simulink model "RGB2YCbCr"  (R2018a)
settings: Solver=VariableStepAuto  StartTime=0.0  StopTime=inf  RelTol=1e-3
InitFcn:
  | height = str2num(get_param([bdroot, '/Image Properties'], 'height'));
  | width = str2num(get_param([bdroot, '/Image Properties'], 'width'));
  | I = imresize(eval(get_param([bdroot, '/Image Properties'], 'image')), [(height) (width)]);
  | I = padarray(I, [1 1], 'replicate');
  | % Change input array to RBG
  | inarray = uint32(double(I(:,:,1))*2^16 + double(I(:,:,3))*2^8 + double(I(:,:,2)));
StopFcn:
  | Out = permute(reshape(simout, [3 width height]), [3 2 1]);
  | imtool(Out);
libraries: xbsIndex_r4 x82, hdlsllib x8, simulink x5, dspsrcs4 x1
settings Model: Creator=rgb11127  LastModifiedBy=Adrian

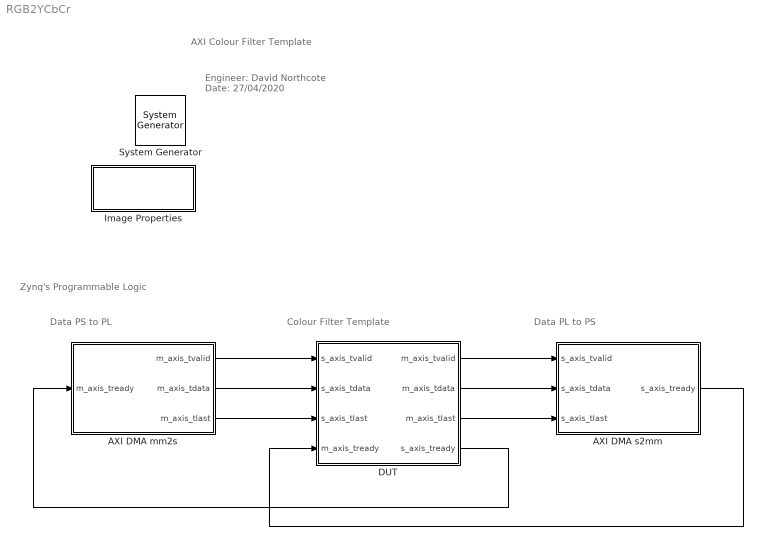
== system RGB2YCbCr ==
  note: Engineer:	David Northcote
      | Date:		27/04/2020
  note: AXI Colour Filter Template
  note: Zynq's Programmable Logic
  note: Data PS to PL
  note: Colour Filter Template
  note: Data PL to PS
  " System Generator" : xbsIndex_r4/ System Generator  Tag=genX  xilinxfamily=zynq  part=xc7z020  speed=-1  package=clg400  synthesis_tool=Vivado  clock_wrapper=Clock Enables  directory=colour_IP  proj_type=Vivado  Synth_file=Vivado Synthesis Defaults  Impl_file=Vivado Implementation Defaults  testbench=off  simulink_period=1/100e6  sysclk_period=10  dcm_input_clock_period=10  incr_netlist=off  trim_vbits=Everywhere in SubSystem  dbl_ovrd=According to Block Masks  core_generation=According to Block Masks  run_coregen=off  deprecated_control=off  eval_field=0  block_type=sysgen
  AXI DMA mm2s : Subsystem  mask{data=inarray, rate=1/100e6, bits=32}
      mask prompts: data "Input Data:"; rate "Sample Time:"; bits "Wordlength:"
      mask init:
      | [height, width] = size(data);
      | 
      | totalsize = height*width;
      | 
      | input = reshape(data', [height*width, 1]);
      | 
      | word = str2num(get_param(gcb, 'bits'));
      mask TypeOptions bits: 8 | 16 | 24 | 32 | 40 | 48 | 56 | 64 | 72 | 80 | 88 | 96 | 104 | 112 | 120 | 128
      mask DialogControl DescGroupVar Prompt: AXI DMA mm2s
      mask DialogControl DescTextVar Prompt: This block simulates an AXI-Stream input from an AXI DMA.
      mask DialogControl ParameterGroupVar Prompt: Main
  AXI DMA s2mm : Subsystem  mask{totalsize=height*width, d=0, rate=1/100e6}
      mask prompts: totalsize "Buffer Size:"; d "Frame Number:"; rate "Sample Rate:"
      mask DialogControl DescGroupVar Prompt: AXI DMA s2mm
      mask DialogControl DescTextVar Prompt: This block simulates an AXI-Stream output to an AXI DMA.
      mask DialogControl ParameterGroupVar Prompt: Main
  DUT : Subsystem
  Image Properties : Subsystem  mask{image=imread('peppers.png'), height=384, width=512}
      mask prompts: image "Input Image:"; height "Image Height:"; width "Image Width:"
      mask init:
      | str = [width];
      mask DialogControl DescGroupVar Prompt: Image Properties
      mask DialogControl DescTextVar Prompt: Set the image and its size using the parameters below.
      mask DialogControl ParameterGroupVar Prompt: Main
      mask Display: disp('Properties')
  wires:
  AXI DMA mm2s/1(m_axis_tvalid) -> DUT/1(s_axis_tvalid)
  AXI DMA mm2s/2(m_axis_tdata) -> DUT/2(s_axis_tdata)
  AXI DMA mm2s/3(m_axis_tlast) -> DUT/3(s_axis_tlast)
  DUT/1(m_axis_tvalid) -> AXI DMA s2mm/1(s_axis_tvalid)
  DUT/2(m_axis_tdata) -> AXI DMA s2mm/2(s_axis_tdata)
  DUT/3(m_axis_tlast) -> AXI DMA s2mm/3(s_axis_tlast)
  DUT/4(s_axis_tready) -> AXI DMA mm2s/1(m_axis_tready)
  AXI DMA s2mm/1(s_axis_tready) -> DUT/4(m_axis_tready)

== system RGB2YCbCr/AXI DMA mm2s ==
  m_axis_tready : Inport
  Compare To Constant : simulink/Logic and Bit Operations/Compare To Constant  relop===  const=totalsize-1  OutDataTypeStr=boolean
  Data Type Conversion : DataTypeConversion  OutDataTypeStr=fixdt(0, word, 0)  ConvertRealWorld=Stored Integer (SI)
  HDL Counter : hdlsllib/Sources/HDL Counter  CountType=Count limited  CountInit=0  CountStep=1  CountMax=totalsize-1  CountFromType=Initial value  CountFrom=0  CountResetPort=off  CountLoadPort=off  CountEnbPort=on  CountDirPort=off  CountDataType=Unsigned  CountWordLen=ceil(log2(totalsize))  CountFracLen=0  CountSampTime=1
      settings: SourceProductBaseCode=HD
  Master AXI-Stream FIFO : Subsystem  mask{sdepth=32}
      mask prompts: sdepth "FIFO Depth:"
      mask init:
      | set_param([gcb, '/HDL FIFO TDATA'], 'fifo_size', get_param(gcb, 'sdepth'));
      | set_param([gcb, '/HDL FIFO TLAST'], 'fifo_size', get_param(gcb, 'sdepth'));
      | 
      | set_param([gcb, '/Compare To Constant'], 'const', num2str(floor(str2num(get_param(gcb, 'sdepth'))/2)));
      mask TypeOptions sdepth: 16 | 32 | 64 | 128 | 256 | 512 | 1024 | 2048 | 4096 | 8192 | 16384 | 32768
      mask DialogControl DescGroupVar Prompt: Master AXI-Stream FIFO
      mask DialogControl DescTextVar Prompt: A custom AXI-Stream FIFO for sending data to other architectures.
      mask DialogControl ParameterGroupVar Prompt: Main
  Synchronous Source : Subsystem  TreatAsAtomicUnit=on
  m_axis_tvalid : Outport
  m_axis_tdata : Outport  Port=2
  m_axis_tlast : Outport  Port=3
  wires:
  m_axis_tready/1 -> Master AXI-Stream FIFO/4(m_axis_tready)
  Master AXI-Stream FIFO/1(m_axis_tvalid) -> m_axis_tvalid/1
  Master AXI-Stream FIFO/2(m_axis_tdata) -> m_axis_tdata/1
  Master AXI-Stream FIFO/3(m_axis_tlast) -> m_axis_tlast/1
  HDL Counter/1 -> Compare To Constant/1
  Compare To Constant/1 -> Master AXI-Stream FIFO/3(s_axis_tlast)
  Master AXI-Stream FIFO/4(s_axis_tready) -> Synchronous Source/Enable, Master AXI-Stream FIFO/1(s_axis_tvalid), HDL Counter/1
  Synchronous Source/1(Data) -> Data Type Conversion/1
  Data Type Conversion/1 -> Master AXI-Stream FIFO/2(s_axis_tdata)

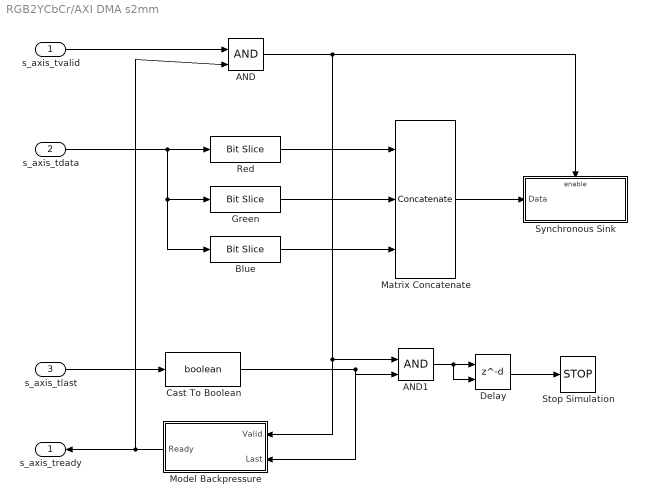
== system RGB2YCbCr/AXI DMA s2mm ==
  s_axis_tvalid : Inport
  s_axis_tdata : Inport  Port=2
  s_axis_tlast : Inport  Port=3
  AND : Logic  IconShape=distinctive  AllPortsSameDT=off  OutDataTypeStr=boolean
  AND1 : Logic  IconShape=distinctive  AllPortsSameDT=off  OutDataTypeStr=boolean
  Blue : hdlsllib/Logic and Bit Operations/Bit Slice  lidx=15  ridx=8
  Cast To Boolean : DataTypeConversion  OutDataTypeStr=boolean
  Delay : Delay  DelayLength=d  ShowEnablePort=on
      settings: InputPortMap=u0,e6
  Green : hdlsllib/Logic and Bit Operations/Bit Slice  lidx=7  ridx=0
  Matrix Concatenate : Concatenate  NumInputs=3  Mode=Multidimensional array
  Model Backpressure : Subsystem
  Red : hdlsllib/Logic and Bit Operations/Bit Slice  lidx=23  ridx=16
  Stop Simulation : Stop
  Synchronous Sink : Subsystem  TreatAsAtomicUnit=on
  s_axis_tready : Outport
  wires:
  s_axis_tvalid/1 -> AND/1
  s_axis_tlast/1 -> Cast To Boolean/1
  AND/1 -> AND1/1, Model Backpressure/1(Valid), Synchronous Sink/Enable
  Model Backpressure/1(Ready) -> AND/2, s_axis_tready/1
  Delay/1 -> Stop Simulation/1
  AND1/1 -> Delay/2, Delay/1
  Cast To Boolean/1 -> Model Backpressure/2(Last), AND1/2
  Matrix Concatenate/1 -> Synchronous Sink/1(Data)
  Red/1 -> Matrix Concatenate/1
  Green/1 -> Matrix Concatenate/2
  Blue/1 -> Matrix Concatenate/3
  s_axis_tdata/1 -> Blue/1, Green/1, Red/1

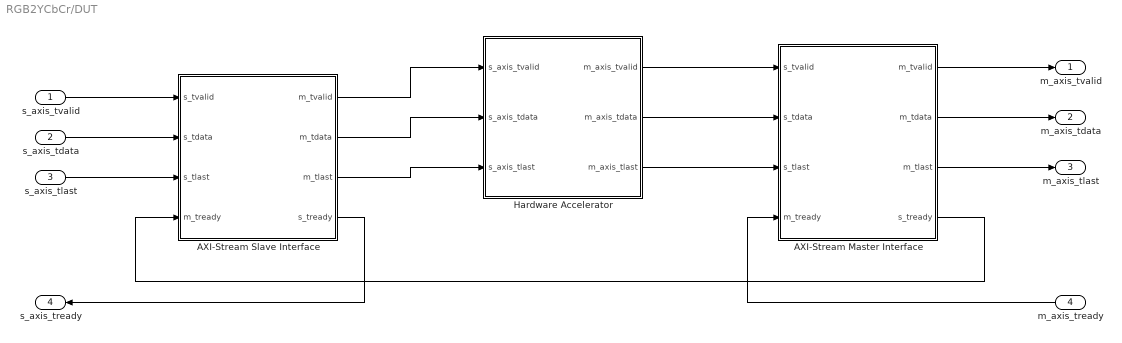
== system RGB2YCbCr/DUT ==
  s_axis_tvalid : Inport
  s_axis_tdata : Inport  Port=2
  s_axis_tlast : Inport  Port=3
  m_axis_tready : Inport  Port=4
  AXI-Stream Master Interface : Subsystem  mask{sdepth=256, rate=1/100e6}
      mask prompts: sdepth "FIFO Depth:"; rate "Sample Rate:"
      mask init:
      | set_param([gcb, '/FIFO TLAST'], 'depth', get_param(gcb, 'sdepth')); 
      | set_param([gcb, '/FIFO TDATA'], 'depth', get_param(gcb, 'sdepth')); 
      | 
      | switch get_param(gcb, 'sdepth')
      |     case '16'
      |         depth = 16;
      |     case '32'
      |         depth = 32;
      |     case '64'
      |         depth = 64;
      |     case '128'
      |         depth = 128;
      |     case '256'
      |         depth = 256;
      |     case '512'
      |         depth = 512;
      |     case '1K'
      |         depth = 1024;
      |     case '2K'
      |         depth = 2048;
      |     case '4K'
      |         depth = 4096;
      |     case '8K'
      |         depth = 8192;
      |     case '16K'
      |         depth = 16384;
      |     case '32K'
      |         depth = 32768;
      |     case '64K'
      |         depth = 65536;
      |     case '128K'
      |         depth = 131072;
      |     case '256K'
      |         depth = 262144;
      |     case '512K'
      |         depth = 524288;
      |     case '1M'
      |         depth = 1048576;
      |     case '2M'
      |         depth = 2097152;
      |     case '4M'
      |         depth = 4194304;
      |     otherwise
      |         depth = 16;
      | end
      mask TypeOptions sdepth: 16 | 32 | 64 | 128 | 256 | 512 | 1K | 2K | 4K | 8K | 16K | 32K | 64K | 128K | 256K | 512K | 1M | 2M | 4M
      mask DialogControl DescGroupVar Prompt: AXI-Stream Master Interface
      mask DialogControl DescTextVar Prompt: System generator gateway and FIFO for the AXI-Stream master interface.
      mask DialogControl ParameterGroupVar Prompt: Main
  AXI-Stream Slave Interface : Subsystem  mask{sdepth=256, sbits=32, rate=1/100e6}
      mask prompts: sdepth "FIFO Depth:"; sbits "TData Width:"; rate "Sample Rate:"
      mask init:
      | set_param([gcb, '/FIFO TLAST'], 'depth', get_param(gcb, 'sdepth')); 
      | set_param([gcb, '/FIFO TDATA'], 'depth', get_param(gcb, 'sdepth')); 
      | 
      | bits = str2num(get_param(gcb, 'sbits'));
      mask TypeOptions sdepth: 16 | 32 | 64 | 128 | 256 | 512 | 1K | 2K | 4K | 8K | 16K | 32K | 64K | 128K | 256K | 512K | 1M | 2M | 4M
      mask TypeOptions sbits: 8 | 16 | 24 | 32 | 40 | 48 | 56 | 64 | 72 | 80 | 88 | 96 | 104 | 112 | 120 | 128
      mask DialogControl DescGroupVar Prompt: AXI-Stream Slave Interface
      mask DialogControl DescTextVar Prompt: System generator gateway and FIFO for the AXI-Stream slave interface.
      mask DialogControl ParameterGroupVar Prompt: Main
  Hardware Accelerator : Subsystem
  m_axis_tvalid : Outport
  m_axis_tdata : Outport  Port=2
  m_axis_tlast : Outport  Port=3
  s_axis_tready : Outport  Port=4
  wires:
  s_axis_tvalid/1 -> AXI-Stream Slave Interface/1(s_tvalid)
  s_axis_tdata/1 -> AXI-Stream Slave Interface/2(s_tdata)
  s_axis_tlast/1 -> AXI-Stream Slave Interface/3(s_tlast)
  AXI-Stream Slave Interface/4(s_tready) -> s_axis_tready/1
  AXI-Stream Master Interface/1(m_tvalid) -> m_axis_tvalid/1
  AXI-Stream Master Interface/2(m_tdata) -> m_axis_tdata/1
  AXI-Stream Master Interface/3(m_tlast) -> m_axis_tlast/1
  m_axis_tready/1 -> AXI-Stream Master Interface/4(m_tready)
  Hardware Accelerator/1(m_axis_tvalid) -> AXI-Stream Master Interface/1(s_tvalid)
  Hardware Accelerator/2(m_axis_tdata) -> AXI-Stream Master Interface/2(s_tdata)
  Hardware Accelerator/3(m_axis_tlast) -> AXI-Stream Master Interface/3(s_tlast)
  AXI-Stream Slave Interface/1(m_tvalid) -> Hardware Accelerator/1(s_axis_tvalid)
  AXI-Stream Slave Interface/2(m_tdata) -> Hardware Accelerator/2(s_axis_tdata)
  AXI-Stream Slave Interface/3(m_tlast) -> Hardware Accelerator/3(s_axis_tlast)
  AXI-Stream Master Interface/4(s_tready) -> AXI-Stream Slave Interface/4(m_tready)

== system RGB2YCbCr/Image Properties ==

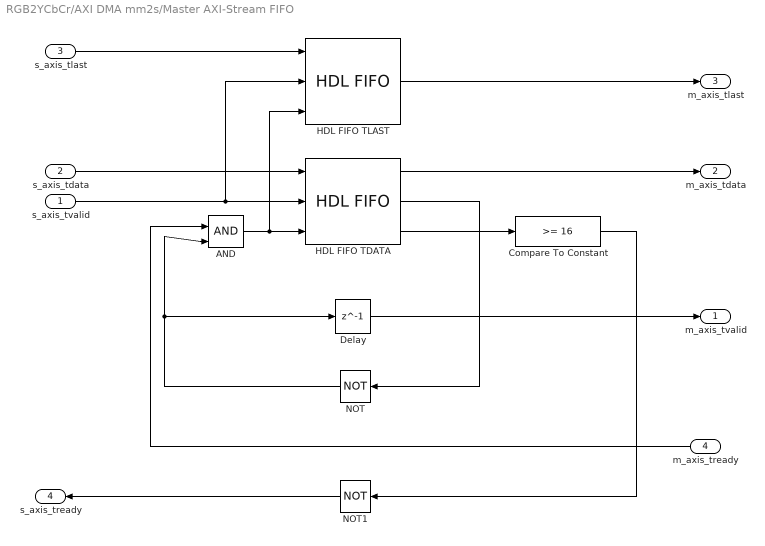
== system RGB2YCbCr/AXI DMA mm2s/Master AXI-Stream FIFO ==
  s_axis_tvalid : Inport
  s_axis_tdata : Inport  Port=2
  s_axis_tlast : Inport  Port=3
  m_axis_tready : Inport  Port=4
  AND : Logic  IconShape=distinctive  AllPortsSameDT=off  OutDataTypeStr=boolean
  Compare To Constant : simulink/Logic and Bit Operations/Compare To Constant  relop=>=  const=16  OutDataTypeStr=boolean
  Delay : Delay  DelayLength=1
  HDL FIFO TDATA : hdlsllib/HDL RAMs/HDL FIFO  fifo_size=32  ratio=1  push_msg=Error  pop_msg=Error  show_empty=on  show_full=off  show_num=on
      settings: SourceProductName=HDL Coder  SourceProductBaseCode=HD
  HDL FIFO TLAST : hdlsllib/HDL RAMs/HDL FIFO  fifo_size=32  ratio=1  push_msg=Error  pop_msg=Error  show_empty=off  show_full=off  show_num=off
      settings: SourceProductName=HDL Coder  SourceProductBaseCode=HD
  NOT : Logic  Operator=NOT  IconShape=distinctive  AllPortsSameDT=off  OutDataTypeStr=boolean
  NOT1 : Logic  Operator=NOT  IconShape=distinctive  AllPortsSameDT=off  OutDataTypeStr=boolean
  m_axis_tvalid : Outport
  m_axis_tdata : Outport  Port=2
  m_axis_tlast : Outport  Port=3
  s_axis_tready : Outport  Port=4
  wires:
  HDL FIFO TDATA/3 -> Compare To Constant/1
  Delay/1 -> m_axis_tvalid/1
  s_axis_tlast/1 -> HDL FIFO TLAST/1
  m_axis_tready/1 -> AND/1
  AND/1 -> HDL FIFO TLAST/3, HDL FIFO TDATA/3
  HDL FIFO TDATA/2 -> NOT/1
  NOT/1 -> Delay/1, AND/2
  HDL FIFO TLAST/1 -> m_axis_tlast/1
  HDL FIFO TDATA/1 -> m_axis_tdata/1
  Compare To Constant/1 -> NOT1/1
  NOT1/1 -> s_axis_tready/1
  s_axis_tdata/1 -> HDL FIFO TDATA/1
  s_axis_tvalid/1 -> HDL FIFO TLAST/2, HDL FIFO TDATA/2

== system RGB2YCbCr/AXI DMA mm2s/Synchronous Source ==
  Enable : EnablePort
  Signal From Workspace : dspsrcs4/Signal From Workspace  X=input  Ts=rate  nsamps=1  OutputAfterFinalValue=Cyclic repetition  ignoreOrWarnInputAndFrameLengths=off  OutputFrames=off
  Data : Outport
  wires:
  Signal From Workspace/1 -> Data/1

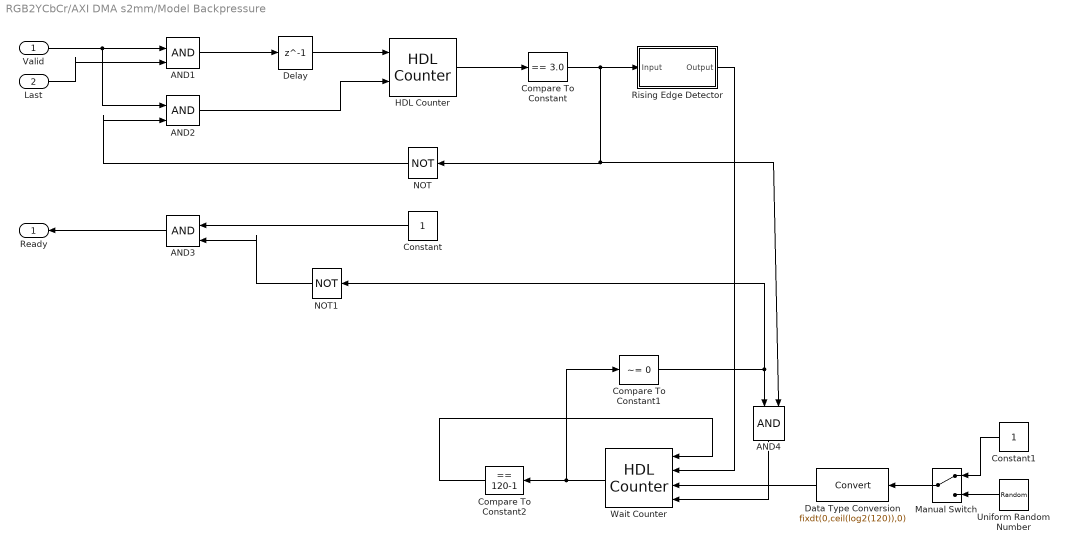
== system RGB2YCbCr/AXI DMA s2mm/Model Backpressure ==
  Valid : Inport
  Last : Inport  Port=2
  AND{1..4} (4 alike) : Logic  IconShape=distinctive  AllPortsSameDT=off  OutDataTypeStr=boolean
  Compare To Constant : simulink/Logic and Bit Operations/Compare To Constant  relop===  const=3.0  OutDataTypeStr=boolean
  Compare To Constant1 : simulink/Logic and Bit Operations/Compare To Constant  relop=~=  const=0  OutDataTypeStr=boolean
  Compare To Constant2 : simulink/Logic and Bit Operations/Compare To Constant  relop===  const=120-1  OutDataTypeStr=boolean
  Constant : Constant  OutDataTypeStr=boolean  SampleTime=rate
  Constant1 : Constant  OutDataTypeStr=fixdt(0, ceil(log2(120)), 0)  SampleTime=rate
  Data Type Conversion : DataTypeConversion  OutDataTypeStr=fixdt(0,ceil(log2(120)),0)
  Delay : Delay  DelayLength=1
  HDL Counter : hdlsllib/Sources/HDL Counter  CountType=Count limited  CountInit=0  CountStep=1  CountMax=totalsize-1  CountFromType=Initial value  CountFrom=0  CountResetPort=on  CountLoadPort=off  CountEnbPort=on  CountDirPort=off  CountDataType=Unsigned  CountWordLen=ceil(log2(totalsize))  CountFracLen=0  CountSampTime=1
      settings: SourceProductBaseCode=HD
  Manual Switch : ManualSwitch
  NOT : Logic  Operator=NOT  IconShape=distinctive  AllPortsSameDT=off  OutDataTypeStr=boolean
  NOT1 : Logic  Operator=NOT  IconShape=distinctive  AllPortsSameDT=off  OutDataTypeStr=boolean
  Rising Edge Detector : Subsystem
  Uniform Random Number : UniformRandomNumber  Minimum=0  Maximum=120-1  Seed=round(rand*10)  SampleTime=rate
  Wait Counter : hdlsllib/Sources/HDL Counter  CountType=Count limited  CountInit=0  CountStep=1  CountMax=120-1  CountFromType=Initial value  CountFrom=0  CountResetPort=on  CountLoadPort=on  CountEnbPort=on  CountDirPort=off  CountDataType=Unsigned  CountWordLen=ceil(log2(120))  CountFracLen=0  CountSampTime=1
      settings: SourceProductBaseCode=HD
  Ready : Outport
  wires:
  AND4/1 -> Wait Counter/4
  Constant/1 -> AND3/1
  Data Type Conversion/1 -> Wait Counter/3
  Delay/1 -> HDL Counter/1
  AND1/1 -> Delay/1
  Last/1 -> AND1/2
  Compare To Constant2/1 -> Wait Counter/1
  NOT/1 -> AND2/2
  Compare To Constant1/1 -> NOT1/1, AND4/1
  HDL Counter/1 -> Compare To Constant/1
  Compare To Constant/1 -> AND4/2, NOT/1, Rising Edge Detector/1(Input)
  NOT1/1 -> AND3/2
  Rising Edge Detector/1(Output) -> Wait Counter/2
  Wait Counter/1 -> Compare To Constant2/1, Compare To Constant1/1
  Valid/1 -> AND2/1, AND1/1
  AND2/1 -> HDL Counter/2
  AND3/1 -> Ready/1
  Uniform Random Number/1 -> Manual Switch/2
  Manual Switch/1 -> Data Type Conversion/1
  Constant1/1 -> Manual Switch/1

== system RGB2YCbCr/AXI DMA s2mm/Synchronous Sink ==
  Data : Inport
  Enable : EnablePort
  To Workspace : ToWorkspace  VariableName=simout  SampleTime=-1
      settings: MaxDataPoints=totalsize
  wires:
  Data/1 -> To Workspace/1

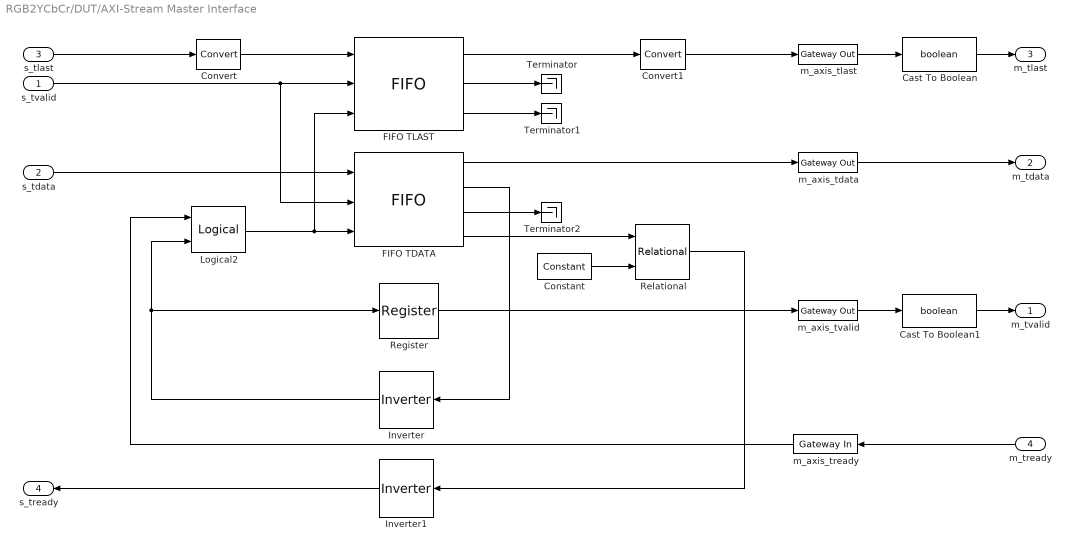
== system RGB2YCbCr/DUT/AXI-Stream Master Interface ==
  s_tvalid : Inport
  s_tdata : Inport  Port=2
  s_tlast : Inport  Port=3
  m_tready : Inport  Port=4
  Cast To Boolean : DataTypeConversion  OutDataTypeStr=boolean
  Cast To Boolean1 : DataTypeConversion  OutDataTypeStr=boolean
  Constant : xbsIndex_r4/Constant  const=floor(depth/2)  gui_display_data_type=Fixed-point  arith_type=Unsigned  n_bits=ceil(log2(depth))  bin_pt=0  preci_type=Single  exp_width=8  frac_width=24  explicit_period=on  period=rate  equ=P=C  opselect=C  inp2=PCIN>>17  opr=+  inp1=P  carry=CIN  dbl_ovrd=off  block_type=constant
  Convert : xbsIndex_r4/Convert  gui_display_data_type=Fixed-point  arith_type=Unsigned  n_bits=1  bin_pt=0  float_type=Single  exp_bits=8  fraction_bits=24  quantization=Truncate  overflow=Wrap  en=off  latency=0  pipeline=off  dbl_ovrd=off  block_type=convert
  Convert1 : xbsIndex_r4/Convert  gui_display_data_type=Boolean  arith_type=Boolean  n_bits=1  bin_pt=0  float_type=Single  exp_bits=8  fraction_bits=24  quantization=Truncate  overflow=Wrap  en=off  latency=0  pipeline=off  dbl_ovrd=off  block_type=convert
  FIFO TDATA : xbsIndex_r4/FIFO  mem_type=Distributed RAM  performance_options=Standard_FIFO  embedded_registers=off  depth=256  percent_nbits=1  rst=off  rst_latency=1  en=off  use_dcount=on  use_percent_full_port=off  use_almost_empty=off  almost_empty_thresh=2  use_almost_full=off  almost_full_thresh=14  explicit_period=off  dbl_ovrd=off  block_type=fifo
  FIFO TLAST : xbsIndex_r4/FIFO  mem_type=Distributed RAM  performance_options=Standard_FIFO  embedded_registers=off  depth=256  percent_nbits=1  rst=off  rst_latency=1  en=off  use_dcount=off  use_percent_full_port=off  use_almost_empty=off  almost_empty_thresh=2  use_almost_full=off  almost_full_thresh=14  explicit_period=off  dbl_ovrd=off  block_type=fifo
  Inverter : xbsIndex_r4/Inverter  en=off  latency=0  dbl_ovrd=off  block_type=inv
  Inverter1 : xbsIndex_r4/Inverter  en=off  latency=0  dbl_ovrd=off  block_type=inv
  Logical2 : xbsIndex_r4/Logical  logical_function=AND  inputs=2  en=off  latency=0  precision=Full  arith_type=Unsigned  n_bits=16  bin_pt=0  align_bp=on  dbl_ovrd=off  block_type=logical
  Register : xbsIndex_r4/Register  init=0  rst=off  en=off  dbl_ovrd=off  block_type=register
  Relational : xbsIndex_r4/Relational  mode=a>=b  op_type=Bool  en=off  latency=0  dbl_ovrd=off  block_type=relational
  Terminator : Terminator
  Terminator1 : Terminator
  Terminator2 : Terminator
  m_axis_tdata : xbsIndex_r4/Gateway Out  inherit_from_input=on  hdl_port=on  rows=1  columns=1  UseAsDAC=off  DACChannel='1'  interface=None  automatic_assignment=on  address_offset=hex2dec('00')  intf_name=''  intf_description=''  timing_constraint=None  locs_specified=off  LOCs={}  io_standard={}  block_type=gatewayout
  m_axis_tlast : xbsIndex_r4/Gateway Out  inherit_from_input=on  hdl_port=on  rows=1  columns=1  UseAsDAC=off  DACChannel='1'  interface=None  automatic_assignment=on  address_offset=hex2dec('00')  intf_name=''  intf_description=''  timing_constraint=None  locs_specified=off  LOCs={}  io_standard={}  block_type=gatewayout
  m_axis_tready : xbsIndex_r4/Gateway In  gui_display_data_type=Boolean  arith_type=Boolean  n_bits=16  bin_pt=14  preci_type=Single  exp_width=8  frac_width=24  rows=1  columns=1  quantization="Round  (unbiased: +/- Inf)"  overflow=Saturate  period=rate  UseAsADC=off  ADCChannel='1'  interface=None  automatic_assignment=on  address_offset=hex2dec('00')  intf_name=''  intf_description=''  default_value=0  timing_constraint=None  locs_specified=off  LOCs={}  io_standard={}  inherit_from_input=off  hdl_port=on  dbl_ovrd=off  block_type=gatewayin
  m_axis_tvalid : xbsIndex_r4/Gateway Out  inherit_from_input=on  hdl_port=on  rows=1  columns=1  UseAsDAC=off  DACChannel='1'  interface=None  automatic_assignment=on  address_offset=hex2dec('00')  intf_name=''  intf_description=''  timing_constraint=None  locs_specified=off  LOCs={}  io_standard={}  block_type=gatewayout
  m_tvalid : Outport
  m_tdata : Outport  Port=2
  m_tlast : Outport  Port=3
  s_tready : Outport  Port=4
  wires:
  Inverter1/1 -> s_tready/1
  Convert/1 -> FIFO TLAST/1
  s_tdata/1 -> FIFO TDATA/1
  s_tlast/1 -> Convert/1
  Logical2/1 -> FIFO TLAST/3, FIFO TDATA/3
  m_tready/1 -> m_axis_tready/1
  Inverter/1 -> Register/1, Logical2/2
  FIFO TDATA/2 -> Inverter/1
  FIFO TDATA/1 -> m_axis_tdata/1
  Register/1 -> m_axis_tvalid/1
  FIFO TLAST/1 -> Convert1/1
  FIFO TLAST/3 -> Terminator1/1
  FIFO TLAST/2 -> Terminator/1
  m_axis_tlast/1 -> Cast To Boolean/1
  m_axis_tdata/1 -> m_tdata/1
  m_axis_tvalid/1 -> Cast To Boolean1/1
  m_axis_tready/1 -> Logical2/1
  FIFO TDATA/3 -> Terminator2/1
  FIFO TDATA/4 -> Relational/1
  Constant/1 -> Relational/2
  Relational/1 -> Inverter1/1
  Convert1/1 -> m_axis_tlast/1
  s_tvalid/1 -> FIFO TDATA/2, FIFO TLAST/2
  Cast To Boolean/1 -> m_tlast/1
  Cast To Boolean1/1 -> m_tvalid/1

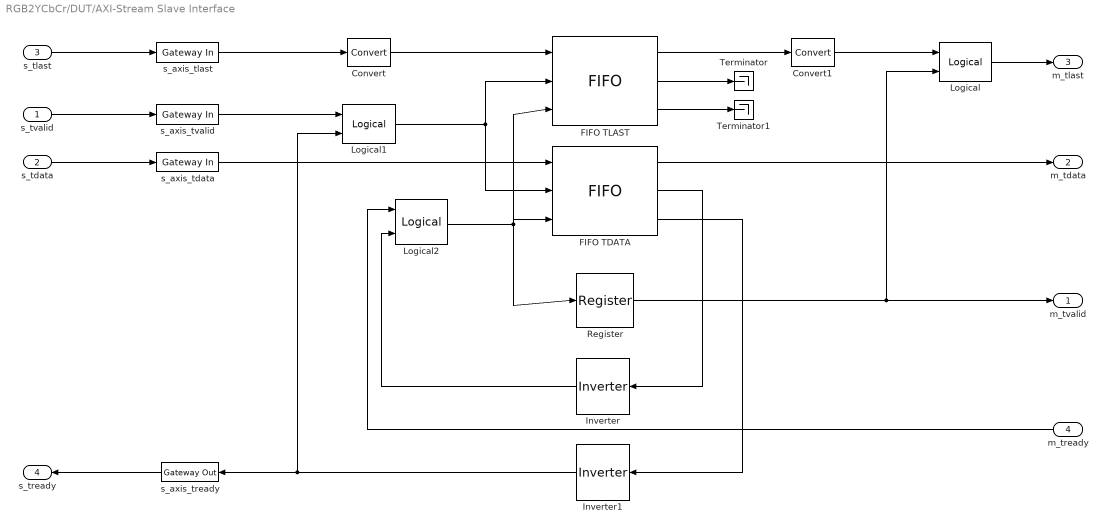
== system RGB2YCbCr/DUT/AXI-Stream Slave Interface ==
  s_tvalid : Inport
  s_tdata : Inport  Port=2
  s_tlast : Inport  Port=3
  m_tready : Inport  Port=4
  Convert : xbsIndex_r4/Convert  gui_display_data_type=Fixed-point  arith_type=Unsigned  n_bits=1  bin_pt=0  float_type=Single  exp_bits=8  fraction_bits=24  quantization=Truncate  overflow=Wrap  en=off  latency=0  pipeline=off  dbl_ovrd=off  block_type=convert
  Convert1 : xbsIndex_r4/Convert  gui_display_data_type=Boolean  arith_type=Boolean  n_bits=1  bin_pt=0  float_type=Single  exp_bits=8  fraction_bits=24  quantization=Truncate  overflow=Wrap  en=off  latency=0  pipeline=off  dbl_ovrd=off  block_type=convert
  FIFO TDATA : xbsIndex_r4/FIFO  mem_type=Distributed RAM  performance_options=Standard_FIFO  embedded_registers=off  depth=256  percent_nbits=1  rst=off  rst_latency=1  en=off  use_dcount=off  use_percent_full_port=off  use_almost_empty=off  almost_empty_thresh=2  use_almost_full=off  almost_full_thresh=14  explicit_period=off  dbl_ovrd=off  block_type=fifo
  FIFO TLAST : xbsIndex_r4/FIFO  mem_type=Distributed RAM  performance_options=Standard_FIFO  embedded_registers=off  depth=256  percent_nbits=1  rst=off  rst_latency=1  en=off  use_dcount=off  use_percent_full_port=off  use_almost_empty=off  almost_empty_thresh=2  use_almost_full=off  almost_full_thresh=14  explicit_period=off  dbl_ovrd=off  block_type=fifo
  Inverter : xbsIndex_r4/Inverter  en=off  latency=0  dbl_ovrd=off  block_type=inv
  Inverter1 : xbsIndex_r4/Inverter  en=off  latency=0  dbl_ovrd=off  block_type=inv
  Logical : xbsIndex_r4/Logical  logical_function=AND  inputs=2  en=off  latency=0  precision=Full  arith_type=Unsigned  n_bits=16  bin_pt=0  align_bp=on  dbl_ovrd=off  block_type=logical
  Logical1 : xbsIndex_r4/Logical  logical_function=AND  inputs=2  en=off  latency=0  precision=Full  arith_type=Unsigned  n_bits=16  bin_pt=0  align_bp=on  dbl_ovrd=off  block_type=logical
  Logical2 : xbsIndex_r4/Logical  logical_function=AND  inputs=2  en=off  latency=0  precision=Full  arith_type=Unsigned  n_bits=16  bin_pt=0  align_bp=on  dbl_ovrd=off  block_type=logical
  Register : xbsIndex_r4/Register  init=0  rst=off  en=off  dbl_ovrd=off  block_type=register
  Terminator : Terminator
  Terminator1 : Terminator
  s_axis_tdata : xbsIndex_r4/Gateway In  gui_display_data_type=Fixed-point  arith_type=Unsigned  n_bits=bits  bin_pt=0  preci_type=Single  exp_width=8  frac_width=24  rows=1  columns=1  quantization="Round  (unbiased: +/- Inf)"  overflow=Saturate  period=rate  UseAsADC=off  ADCChannel='1'  interface=None  automatic_assignment=on  address_offset=hex2dec('00')  intf_name=''  intf_description=''  default_value=0  timing_constraint=None  locs_specified=off  LOCs={}  io_standard={}  inherit_from_input=off  hdl_port=on  dbl_ovrd=off  block_type=gatewayin
  s_axis_tlast : xbsIndex_r4/Gateway In  gui_display_data_type=Boolean  arith_type=Boolean  n_bits=16  bin_pt=14  preci_type=Single  exp_width=8  frac_width=24  rows=1  columns=1  quantization="Round  (unbiased: +/- Inf)"  overflow=Saturate  period=rate  UseAsADC=off  ADCChannel='1'  interface=None  automatic_assignment=on  address_offset=hex2dec('00')  intf_name=''  intf_description=''  default_value=0  timing_constraint=None  locs_specified=off  LOCs={}  io_standard={}  inherit_from_input=off  hdl_port=on  dbl_ovrd=off  block_type=gatewayin
  s_axis_tready : xbsIndex_r4/Gateway Out  inherit_from_input=on  hdl_port=on  rows=1  columns=1  UseAsDAC=off  DACChannel='1'  interface=None  automatic_assignment=on  address_offset=hex2dec('00')  intf_name=''  intf_description=''  timing_constraint=None  locs_specified=off  LOCs={}  io_standard={}  block_type=gatewayout
  s_axis_tvalid : xbsIndex_r4/Gateway In  gui_display_data_type=Boolean  arith_type=Boolean  n_bits=16  bin_pt=14  preci_type=Single  exp_width=8  frac_width=24  rows=1  columns=1  quantization="Round  (unbiased: +/- Inf)"  overflow=Saturate  period=rate  UseAsADC=off  ADCChannel='1'  interface=None  automatic_assignment=on  address_offset=hex2dec('00')  intf_name=''  intf_description=''  default_value=0  timing_constraint=None  locs_specified=off  LOCs={}  io_standard={}  inherit_from_input=off  hdl_port=on  dbl_ovrd=off  block_type=gatewayin
  m_tvalid : Outport
  m_tdata : Outport  Port=2
  m_tlast : Outport  Port=3
  s_tready : Outport  Port=4
  wires:
  FIFO TLAST/2 -> Terminator/1
  FIFO TLAST/3 -> Terminator1/1
  FIFO TLAST/1 -> Convert1/1
  Register/1 -> m_tvalid/1, Logical/2
  FIFO TDATA/1 -> m_tdata/1
  Logical/1 -> m_tlast/1
  s_tvalid/1 -> s_axis_tvalid/1
  Logical1/1 -> FIFO TLAST/2, FIFO TDATA/2
  s_tlast/1 -> s_axis_tlast/1
  s_tdata/1 -> s_axis_tdata/1
  FIFO TDATA/2 -> Inverter/1
  FIFO TDATA/3 -> Inverter1/1
  Inverter/1 -> Logical2/2
  m_tready/1 -> Logical2/1
  Inverter1/1 -> Logical1/2, s_axis_tready/1
  Logical2/1 -> Register/1, FIFO TLAST/3, FIFO TDATA/3
  s_axis_tlast/1 -> Convert/1
  s_axis_tvalid/1 -> Logical1/1
  s_axis_tdata/1 -> FIFO TDATA/1
  Convert/1 -> FIFO TLAST/1
  Convert1/1 -> Logical/1
  s_axis_tready/1 -> s_tready/1

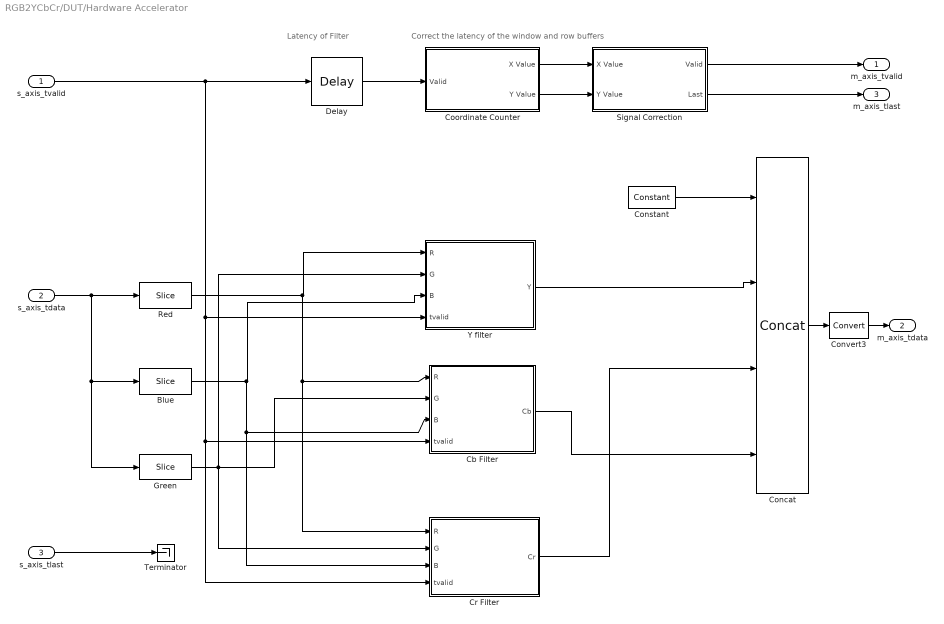
== system RGB2YCbCr/DUT/Hardware Accelerator ==
  note: Correct the latency of the window and row buffers
  note: Latency of Filter
  s_axis_tvalid : Inport
  s_axis_tdata : Inport  Port=2
  s_axis_tlast : Inport  Port=3
  Blue : xbsIndex_r4/Slice  nbits=1  boolean_output=off  mode=Two Bit Locations  bit1=15  base1=LSB of Input  bit0=8  base0=LSB of Input  dbl_ovrd=off  block_type=slice
  Cb Filter : Subsystem
  Concat : xbsIndex_r4/Concat  num_inputs=4  dbl_ovrd=off  block_type=concat
  Constant : xbsIndex_r4/Constant  const=0  gui_display_data_type=Fixed-point  arith_type=Unsigned  n_bits=8  bin_pt=0  preci_type=Single  exp_width=8  frac_width=24  explicit_period=off  period=1  equ=P=C  opselect=C  inp2=PCIN>>17  opr=+  inp1=P  carry=CIN  dbl_ovrd=off  block_type=constant
  Convert3 : xbsIndex_r4/Convert  gui_display_data_type=Fixed-point  arith_type=Unsigned  n_bits=32  bin_pt=0  float_type=Single  exp_bits=8  fraction_bits=24  quantization=Truncate  overflow=Saturate  en=off  latency=1  pipeline=off  dbl_ovrd=off  block_type=convert
  Coordinate Counter : Subsystem
  Cr Filter : Subsystem
  Delay : xbsIndex_r4/Delay  rst=off  infoeditControl=Selection of Reset will increase slice count due to use of real FFs and instead of SRLs  en=off  latency=4  reg_retiming=off  dbl_ovrd=off  block_type=delay
  Green : xbsIndex_r4/Slice  nbits=1  boolean_output=off  mode=Two Bit Locations  bit1=7  base1=LSB of Input  bit0=0  base0=LSB of Input  dbl_ovrd=off  block_type=slice
  Red : xbsIndex_r4/Slice  nbits=1  boolean_output=off  mode=Two Bit Locations  bit1=23  base1=LSB of Input  bit0=16  base0=LSB of Input  dbl_ovrd=off  block_type=slice
  Signal Correction : Subsystem
  Terminator : Terminator
  Y filter : Subsystem
  m_axis_tvalid : Outport
  m_axis_tdata : Outport  Port=2
  m_axis_tlast : Outport  Port=3
  wires:
  s_axis_tlast/1 -> Terminator/1
  s_axis_tdata/1 -> Blue/1, Green/1, Red/1
  Coordinate Counter/1(X Value) -> Signal Correction/1(X Value)
  Coordinate Counter/2(Y Value) -> Signal Correction/2(Y Value)
  Signal Correction/1(Valid) -> m_axis_tvalid/1
  Signal Correction/2(Last) -> m_axis_tlast/1
  s_axis_tvalid/1 -> Cr Filter/4(tvalid), Cb Filter/4(tvalid), Y filter/4(tvalid), Delay/1
  Constant/1 -> Concat/1
  Y filter/1(Y) -> Concat/2
  Cr Filter/1(Cr) -> Concat/3
  Cb Filter/1(Cb) -> Concat/4
  Concat/1 -> Convert3/1
  Convert3/1 -> m_axis_tdata/1
  Delay/1 -> Coordinate Counter/1(Valid)
  Red/1 -> Cr Filter/1(R), Cb Filter/1(R), Y filter/1(R)
  Blue/1 -> Cb Filter/3(B), Cr Filter/3(B), Y filter/3(B)
  Green/1 -> Cr Filter/2(G), Y filter/2(G), Cb Filter/2(G)

== system RGB2YCbCr/AXI DMA s2mm/Model Backpressure/Rising Edge Detector ==
  Input : Inport
  AND3 : Logic  IconShape=distinctive  AllPortsSameDT=off  OutDataTypeStr=boolean
  Delay1 : Delay  DelayLength=1
  NOT1 : Logic  Operator=NOT  IconShape=distinctive  AllPortsSameDT=off  OutDataTypeStr=boolean
  Output : Outport
  wires:
  Input/1 -> AND3/2, NOT1/1
  AND3/1 -> Output/1
  Delay1/1 -> AND3/1
  NOT1/1 -> Delay1/1

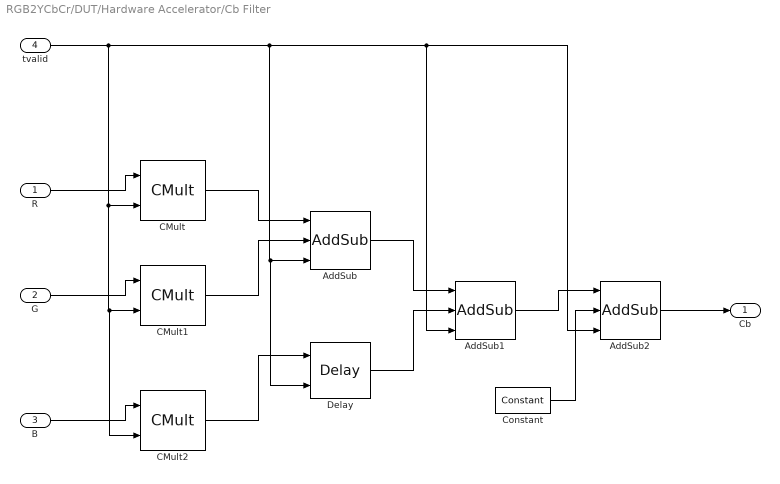
== system RGB2YCbCr/DUT/Hardware Accelerator/Cb Filter ==
  R : Inport
  G : Inport  Port=2
  B : Inport  Port=3
  tvalid : Inport  Port=4
  AddSub : xbsIndex_r4/AddSub  mode=Addition  use_carryin=off  use_carryout=off  en=on  latency=1  precision=Full  arith_type=Unsigned  n_bits=16  bin_pt=14  quantization=Truncate  overflow=Wrap  use_behavioral_HDL=off  hw_selection=Fabric  pipelined=off  dbl_ovrd=off  block_type=addsub
  AddSub1 : xbsIndex_r4/AddSub  mode=Addition  use_carryin=off  use_carryout=off  en=on  latency=1  precision=Full  arith_type=Unsigned  n_bits=16  bin_pt=14  quantization=Truncate  overflow=Wrap  use_behavioral_HDL=off  hw_selection=Fabric  pipelined=off  dbl_ovrd=off  block_type=addsub
  AddSub2 : xbsIndex_r4/AddSub  mode=Addition  use_carryin=off  use_carryout=off  en=on  latency=1  precision=User Defined  arith_type=Unsigned  n_bits=8  bin_pt=0  quantization="Round  (unbiased: +/- Inf)"  overflow=Saturate  use_behavioral_HDL=off  hw_selection=Fabric  pipelined=off  dbl_ovrd=off  block_type=addsub
  CMult : xbsIndex_r4/CMult  const=-0.148  gui_display_data_type=Fixed-point  const_n_bits=16  const_bin_pt=14  float_type=Single  exp_bits=8  fraction_bits=24  en=on  latency=1  precision=Full  arith_type="Signed  (2's comp)"  n_bits=16  bin_pt=14  quantization=Truncate  overflow=Wrap  use_behavioral_HDL=off  mem_type=Distributed RAM  pipeline=off  dbl_ovrd=off  block_type=cmult
  CMult1 : xbsIndex_r4/CMult  const=-0.292  gui_display_data_type=Fixed-point  const_n_bits=16  const_bin_pt=14  float_type=Single  exp_bits=8  fraction_bits=24  en=on  latency=1  precision=Full  arith_type="Signed  (2's comp)"  n_bits=16  bin_pt=14  quantization=Truncate  overflow=Wrap  use_behavioral_HDL=off  mem_type=Distributed RAM  pipeline=off  dbl_ovrd=off  block_type=cmult
  CMult2 : xbsIndex_r4/CMult  const=0.439  gui_display_data_type=Fixed-point  const_n_bits=16  const_bin_pt=14  float_type=Single  exp_bits=8  fraction_bits=24  en=on  latency=1  precision=Full  arith_type="Signed  (2's comp)"  n_bits=16  bin_pt=14  quantization=Truncate  overflow=Wrap  use_behavioral_HDL=off  mem_type=Distributed RAM  pipeline=off  dbl_ovrd=off  block_type=cmult
  Constant : xbsIndex_r4/Constant  const=128  gui_display_data_type=Fixed-point  arith_type=Unsigned  n_bits=16  bin_pt=8  preci_type=Single  exp_width=8  frac_width=24  explicit_period=off  period=1  equ=P=C  opselect=C  inp2=PCIN>>17  opr=+  inp1=P  carry=CIN  dbl_ovrd=off  block_type=constant
  Delay : xbsIndex_r4/Delay  rst=off  infoeditControl=Selection of Reset will increase slice count due to use of real FFs and instead of SRLs  en=on  latency=1  reg_retiming=off  dbl_ovrd=off  block_type=delay
  Cb : Outport
  wires:
  AddSub/1 -> AddSub1/1
  CMult1/1 -> AddSub/2
  CMult2/1 -> Delay/1
  Delay/1 -> AddSub1/2
  CMult/1 -> AddSub/1
  AddSub1/1 -> AddSub2/1
  Constant/1 -> AddSub2/2
  R/1 -> CMult/1
  G/1 -> CMult1/1
  B/1 -> CMult2/1
  AddSub2/1 -> Cb/1
  tvalid/1 -> CMult2/2, CMult1/2, CMult/2, Delay/2, AddSub/3, AddSub1/3, AddSub2/3

== system RGB2YCbCr/DUT/Hardware Accelerator/Coordinate Counter ==
  Valid : Inport
  Constant : xbsIndex_r4/Constant  const=width+1  gui_display_data_type=Fixed-point  arith_type=Unsigned  n_bits=ceil(log2(width+1))  bin_pt=0  preci_type=Single  exp_width=8  frac_width=24  explicit_period=on  period=1/100e6  equ=P=C  opselect=C  inp2=PCIN>>17  opr=+  inp1=P  carry=CIN  dbl_ovrd=off  block_type=constant
  Relational : xbsIndex_r4/Relational  mode=a=b  op_type=Bool  en=off  latency=0  dbl_ovrd=off  block_type=relational
  X Counter : xbsIndex_r4/Counter  cnt_type=Count Limited  cnt_to=width+1  operation=Up  start_count=0  cnt_by_val=1  arith_type=Unsigned  n_bits=ceil(log2(width+2))  bin_pt=0  load_pin=off  rst=off  en=on  explicit_period=off  period=1  use_behavioral_HDL=off  implementation=Fabric  dbl_ovrd=off  block_type=counter
  Y Counter : xbsIndex_r4/Counter  cnt_type=Count Limited  cnt_to=height+1  operation=Up  start_count=0  cnt_by_val=1  arith_type=Unsigned  n_bits=ceil(log2(height+2))  bin_pt=0  load_pin=off  rst=off  en=on  explicit_period=off  period=1  use_behavioral_HDL=off  implementation=Fabric  dbl_ovrd=off  block_type=counter
  X Value : Outport
  Y Value : Outport  Port=2
  wires:
  Constant/1 -> Relational/1
  X Counter/1 -> X Value/1, Relational/2
  Relational/1 -> Y Counter/1
  Valid/1 -> X Counter/1
  Y Counter/1 -> Y Value/1

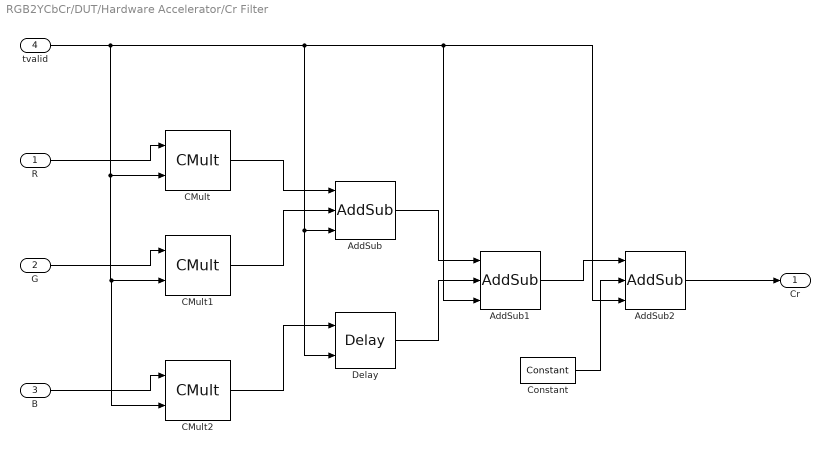
== system RGB2YCbCr/DUT/Hardware Accelerator/Cr Filter ==
  R : Inport
  G : Inport  Port=2
  B : Inport  Port=3
  tvalid : Inport  Port=4
  AddSub : xbsIndex_r4/AddSub  mode=Addition  use_carryin=off  use_carryout=off  en=on  latency=1  precision=Full  arith_type=Unsigned  n_bits=16  bin_pt=14  quantization=Truncate  overflow=Wrap  use_behavioral_HDL=off  hw_selection=Fabric  pipelined=off  dbl_ovrd=off  block_type=addsub
  AddSub1 : xbsIndex_r4/AddSub  mode=Addition  use_carryin=off  use_carryout=off  en=on  latency=1  precision=Full  arith_type=Unsigned  n_bits=16  bin_pt=14  quantization=Truncate  overflow=Wrap  use_behavioral_HDL=off  hw_selection=Fabric  pipelined=off  dbl_ovrd=off  block_type=addsub
  AddSub2 : xbsIndex_r4/AddSub  mode=Addition  use_carryin=off  use_carryout=off  en=on  latency=1  precision=User Defined  arith_type=Unsigned  n_bits=8  bin_pt=0  quantization="Round  (unbiased: +/- Inf)"  overflow=Saturate  use_behavioral_HDL=off  hw_selection=Fabric  pipelined=off  dbl_ovrd=off  block_type=addsub
  CMult : xbsIndex_r4/CMult  const=0.439  gui_display_data_type=Fixed-point  const_n_bits=16  const_bin_pt=14  float_type=Single  exp_bits=8  fraction_bits=24  en=on  latency=1  precision=Full  arith_type="Signed  (2's comp)"  n_bits=16  bin_pt=14  quantization=Truncate  overflow=Wrap  use_behavioral_HDL=off  mem_type=Distributed RAM  pipeline=off  dbl_ovrd=off  block_type=cmult
  CMult1 : xbsIndex_r4/CMult  const=-0.368  gui_display_data_type=Fixed-point  const_n_bits=16  const_bin_pt=14  float_type=Single  exp_bits=8  fraction_bits=24  en=on  latency=1  precision=Full  arith_type="Signed  (2's comp)"  n_bits=16  bin_pt=14  quantization=Truncate  overflow=Wrap  use_behavioral_HDL=off  mem_type=Distributed RAM  pipeline=off  dbl_ovrd=off  block_type=cmult
  CMult2 : xbsIndex_r4/CMult  const=-0.071  gui_display_data_type=Fixed-point  const_n_bits=16  const_bin_pt=14  float_type=Single  exp_bits=8  fraction_bits=24  en=on  latency=1  precision=Full  arith_type="Signed  (2's comp)"  n_bits=16  bin_pt=14  quantization=Truncate  overflow=Wrap  use_behavioral_HDL=off  mem_type=Distributed RAM  pipeline=off  dbl_ovrd=off  block_type=cmult
  Constant : xbsIndex_r4/Constant  const=128  gui_display_data_type=Fixed-point  arith_type=Unsigned  n_bits=16  bin_pt=8  preci_type=Single  exp_width=8  frac_width=24  explicit_period=off  period=1  equ=P=C  opselect=C  inp2=PCIN>>17  opr=+  inp1=P  carry=CIN  dbl_ovrd=off  block_type=constant
  Delay : xbsIndex_r4/Delay  rst=off  infoeditControl=Selection of Reset will increase slice count due to use of real FFs and instead of SRLs  en=on  latency=1  reg_retiming=off  dbl_ovrd=off  block_type=delay
  Cr : Outport
  wires:
  Constant/1 -> AddSub2/2
  Delay/1 -> AddSub1/2
  CMult/1 -> AddSub/1
  CMult1/1 -> AddSub/2
  CMult2/1 -> Delay/1
  AddSub/1 -> AddSub1/1
  AddSub1/1 -> AddSub2/1
  R/1 -> CMult/1
  G/1 -> CMult1/1
  B/1 -> CMult2/1
  AddSub2/1 -> Cr/1
  tvalid/1 -> CMult2/2, CMult1/2, CMult/2, Delay/2, AddSub/3, AddSub1/3, AddSub2/3

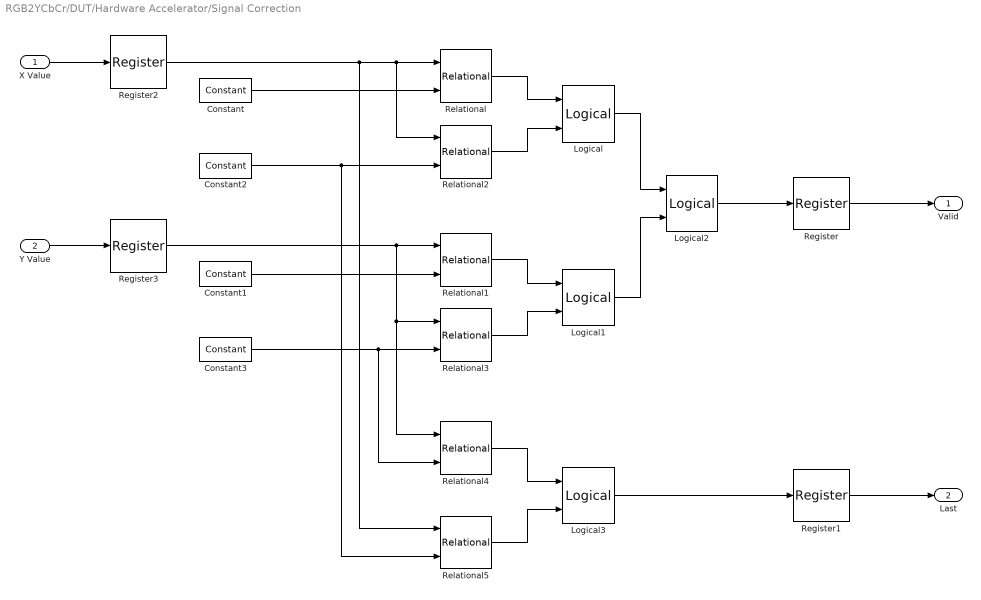
== system RGB2YCbCr/DUT/Hardware Accelerator/Signal Correction ==
  X Value : Inport
  Y Value : Inport  Port=2
  Constant : xbsIndex_r4/Constant  const=1  gui_display_data_type=Fixed-point  arith_type=Unsigned  n_bits=ceil(log2(width+1))  bin_pt=0  preci_type=Single  exp_width=8  frac_width=24  explicit_period=on  period=1/100e6  equ=P=C  opselect=C  inp2=PCIN>>17  opr=+  inp1=P  carry=CIN  dbl_ovrd=off  block_type=constant
  Constant1 : xbsIndex_r4/Constant  const=1  gui_display_data_type=Fixed-point  arith_type=Unsigned  n_bits=ceil(log2(height+1))  bin_pt=0  preci_type=Single  exp_width=8  frac_width=24  explicit_period=on  period=1/100e6  equ=P=C  opselect=C  inp2=PCIN>>17  opr=+  inp1=P  carry=CIN  dbl_ovrd=off  block_type=constant
  Constant2 : xbsIndex_r4/Constant  const=width  gui_display_data_type=Fixed-point  arith_type=Unsigned  n_bits=ceil(log2(width+1))  bin_pt=0  preci_type=Single  exp_width=8  frac_width=24  explicit_period=on  period=1/100e6  equ=P=C  opselect=C  inp2=PCIN>>17  opr=+  inp1=P  carry=CIN  dbl_ovrd=off  block_type=constant
  Constant3 : xbsIndex_r4/Constant  const=height  gui_display_data_type=Fixed-point  arith_type=Unsigned  n_bits=ceil(log2(height+1))  bin_pt=0  preci_type=Single  exp_width=8  frac_width=24  explicit_period=on  period=1/100e6  equ=P=C  opselect=C  inp2=PCIN>>17  opr=+  inp1=P  carry=CIN  dbl_ovrd=off  block_type=constant
  Logical{,1..3} (4 alike) : xbsIndex_r4/Logical  logical_function=AND  inputs=2  en=off  latency=0  precision=Full  arith_type=Unsigned  n_bits=16  bin_pt=0  align_bp=on  dbl_ovrd=off  block_type=logical
  Register{,1..3} (4 alike) : xbsIndex_r4/Register  init=0  rst=off  en=off  dbl_ovrd=off  block_type=register
  Relational : xbsIndex_r4/Relational  mode=a>=b  op_type=Bool  en=off  latency=0  dbl_ovrd=off  block_type=relational
  Relational1 : xbsIndex_r4/Relational  mode=a>=b  op_type=Bool  en=off  latency=0  dbl_ovrd=off  block_type=relational
  Relational2 : xbsIndex_r4/Relational  mode=a<=b  op_type=Bool  en=off  latency=0  dbl_ovrd=off  block_type=relational
  Relational3 : xbsIndex_r4/Relational  mode=a<=b  op_type=Bool  en=off  latency=0  dbl_ovrd=off  block_type=relational
  Relational4 : xbsIndex_r4/Relational  mode=a=b  op_type=Bool  en=off  latency=0  dbl_ovrd=off  block_type=relational
  Relational5 : xbsIndex_r4/Relational  mode=a=b  op_type=Bool  en=off  latency=0  dbl_ovrd=off  block_type=relational
  Valid : Outport
  Last : Outport  Port=2
  wires:
  Constant/1 -> Relational/2
  Constant1/1 -> Relational1/2
  Constant2/1 -> Relational5/2, Relational2/2
  X Value/1 -> Register2/1
  Relational2/1 -> Logical/2
  Relational/1 -> Logical/1
  Y Value/1 -> Register3/1
  Constant3/1 -> Relational4/2, Relational3/2
  Relational1/1 -> Logical1/1
  Relational3/1 -> Logical1/2
  Logical/1 -> Logical2/1
  Logical1/1 -> Logical2/2
  Logical2/1 -> Register/1
  Register/1 -> Valid/1
  Relational4/1 -> Logical3/1
  Relational5/1 -> Logical3/2
  Logical3/1 -> Register1/1
  Register1/1 -> Last/1
  Register2/1 -> Relational5/1, Relational/1, Relational2/1
  Register3/1 -> Relational4/1, Relational3/1, Relational1/1

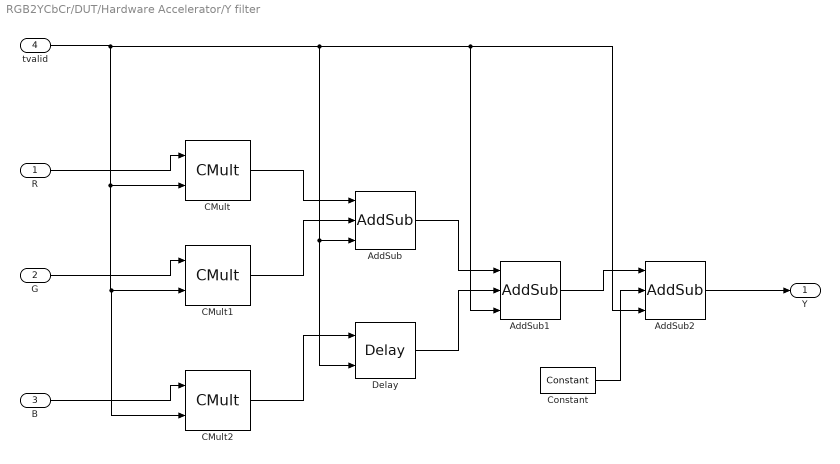
== system RGB2YCbCr/DUT/Hardware Accelerator/Y filter ==
  R : Inport
  G : Inport  Port=2
  B : Inport  Port=3
  tvalid : Inport  Port=4
  AddSub : xbsIndex_r4/AddSub  mode=Addition  use_carryin=off  use_carryout=off  en=on  latency=1  precision=Full  arith_type=Unsigned  n_bits=16  bin_pt=14  quantization=Truncate  overflow=Wrap  use_behavioral_HDL=off  hw_selection=Fabric  pipelined=off  dbl_ovrd=off  block_type=addsub
  AddSub1 : xbsIndex_r4/AddSub  mode=Addition  use_carryin=off  use_carryout=off  en=on  latency=1  precision=Full  arith_type=Unsigned  n_bits=16  bin_pt=14  quantization=Truncate  overflow=Wrap  use_behavioral_HDL=off  hw_selection=Fabric  pipelined=off  dbl_ovrd=off  block_type=addsub
  AddSub2 : xbsIndex_r4/AddSub  mode=Addition  use_carryin=off  use_carryout=off  en=on  latency=1  precision=User Defined  arith_type=Unsigned  n_bits=8  bin_pt=0  quantization="Round  (unbiased: +/- Inf)"  overflow=Saturate  use_behavioral_HDL=off  hw_selection=Fabric  pipelined=off  dbl_ovrd=off  block_type=addsub
  CMult : xbsIndex_r4/CMult  const=0.257  gui_display_data_type=Fixed-point  const_n_bits=16  const_bin_pt=14  float_type=Single  exp_bits=8  fraction_bits=24  en=on  latency=1  precision=Full  arith_type="Signed  (2's comp)"  n_bits=16  bin_pt=14  quantization=Truncate  overflow=Wrap  use_behavioral_HDL=off  mem_type=Distributed RAM  pipeline=off  dbl_ovrd=off  block_type=cmult
  CMult1 : xbsIndex_r4/CMult  const=0.504  gui_display_data_type=Fixed-point  const_n_bits=16  const_bin_pt=14  float_type=Single  exp_bits=8  fraction_bits=24  en=on  latency=1  precision=Full  arith_type="Signed  (2's comp)"  n_bits=16  bin_pt=14  quantization=Truncate  overflow=Wrap  use_behavioral_HDL=off  mem_type=Distributed RAM  pipeline=off  dbl_ovrd=off  block_type=cmult
  CMult2 : xbsIndex_r4/CMult  const=0.098  gui_display_data_type=Fixed-point  const_n_bits=16  const_bin_pt=14  float_type=Single  exp_bits=8  fraction_bits=24  en=on  latency=1  precision=Full  arith_type="Signed  (2's comp)"  n_bits=16  bin_pt=14  quantization=Truncate  overflow=Wrap  use_behavioral_HDL=off  mem_type=Distributed RAM  pipeline=off  dbl_ovrd=off  block_type=cmult
  Constant : xbsIndex_r4/Constant  const=16  gui_display_data_type=Fixed-point  arith_type=Unsigned  n_bits=16  bin_pt=11  preci_type=Single  exp_width=8  frac_width=24  explicit_period=off  period=1  equ=P=C  opselect=C  inp2=PCIN>>17  opr=+  inp1=P  carry=CIN  dbl_ovrd=off  block_type=constant
  Delay : xbsIndex_r4/Delay  rst=off  infoeditControl=Selection of Reset will increase slice count due to use of real FFs and instead of SRLs  en=on  latency=1  reg_retiming=off  dbl_ovrd=off  block_type=delay
  Y : Outport
  wires:
  R/1 -> CMult/1
  G/1 -> CMult1/1
  B/1 -> CMult2/1
  CMult/1 -> AddSub/1
  CMult1/1 -> AddSub/2
  AddSub/1 -> AddSub1/1
  AddSub1/1 -> AddSub2/1
  AddSub2/1 -> Y/1
  Constant/1 -> AddSub2/2
  CMult2/1 -> Delay/1
  Delay/1 -> AddSub1/2
  tvalid/1 -> Delay/2, AddSub/3, AddSub1/3, AddSub2/3, CMult2/2, CMult1/2, CMult/2
